simulink model "Grading_SL_Topic2"  (R2019a)
settings: Solver=FixedStepDiscrete  StartTime=0.0  StopTime=10.0  RelTol=1e-3
settings Model: Creator=Raouf  LastModifiedBy=Raouf
settings OptimizationCC: DefaultParameterBehavior=Inlined  EnhancedBackFolding=on  PassReuseOutputArgsAs=Individual arguments  OptimizeBlockOrder=speed  DifferentSizesBufferReuse=on  OptimizationCustomize=off
settings DebuggingCC: ParameterTunabilityLossMsg=error
settings SFSimCC: MATLABDynamicMemAlloc=off
settings RTWCC: SystemTargetFile=ert.tlc  GenCodeOnly=on  TemplateMakefile=ert_default_tmf  GenerateReport=on  IncludeHyperlinkInReport=on  LaunchReport=on  GenerateTraceInfo=on  GenerateTraceReport=on  GenerateTraceReportSl=on  GenerateTraceReportSf=on  GenerateTraceReportEml=on
settings CodeAppCC: ForceParamTrailComments=on  IgnoreCustomStorageClasses=off  OperatorAnnotations=on  SimulinkDataObjDesc=on  SFDataObjDesc=on  InsertBlockDesc=on
settings ERTTargetCC: TargetLangStandard=C99 (ISO)  GenerateSampleERTMain=on  InlinedParameterPlacement=NonHierarchical  ERTCustomFileTemplate=example_file_process.tlc

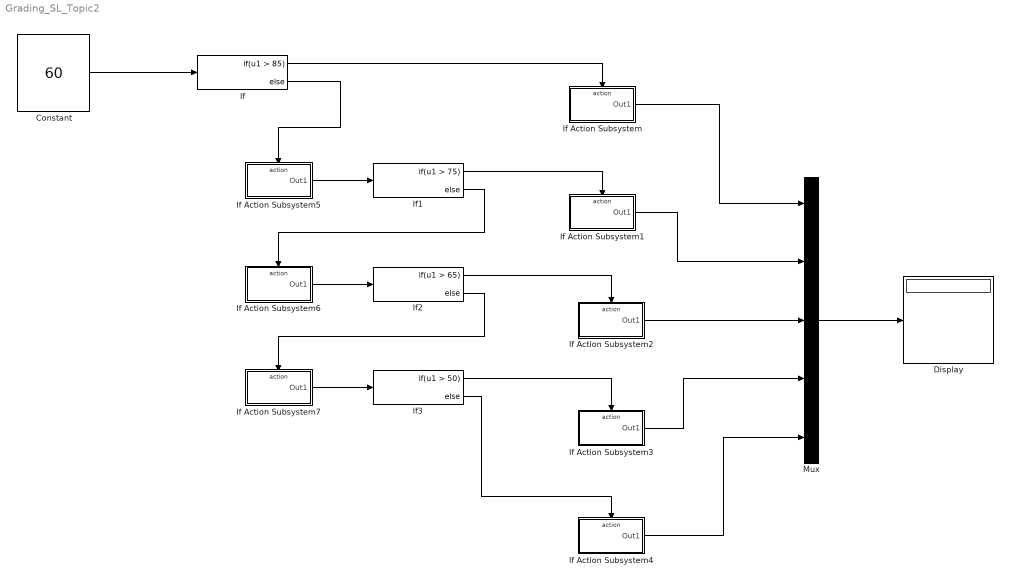
== system Grading_SL_Topic2 ==
  Constant : Constant  Value=60
  Display : Display
  If : If  IfExpression=u1 > 85
  If Action Subsystem : Subsystem  TreatAsAtomicUnit=on
  If Action Subsystem1 : Subsystem  TreatAsAtomicUnit=on
  If Action Subsystem2 : Subsystem  TreatAsAtomicUnit=on
  If Action Subsystem3 : Subsystem  TreatAsAtomicUnit=on
  If Action Subsystem4 : Subsystem  TreatAsAtomicUnit=on
  If Action Subsystem5 : Subsystem  TreatAsAtomicUnit=on
  If Action Subsystem6 : Subsystem  TreatAsAtomicUnit=on
  If Action Subsystem7 : Subsystem  TreatAsAtomicUnit=on
  If1 : If  IfExpression=u1 > 75
  If2 : If  IfExpression=u1 > 65
  If3 : If  IfExpression=u1 > 50
  Mux : Mux  Inputs=5
  wires:
  Constant/1 -> If/1
  If/1 -> If Action Subsystem/Action
  If1/1 -> If Action Subsystem1/Action
  If2/1 -> If Action Subsystem2/Action
  If3/1 -> If Action Subsystem3/Action
  If3/2 -> If Action Subsystem4/Action
  If Action Subsystem/1(Out1) -> Mux/1
  If Action Subsystem1/1(Out1) -> Mux/2
  If Action Subsystem2/1(Out1) -> Mux/3
  If Action Subsystem3/1(Out1) -> Mux/4
  If Action Subsystem4/1(Out1) -> Mux/5
  Mux/1 -> Display/1
  If/2 -> If Action Subsystem5/Action
  If Action Subsystem5/1(Out1) -> If1/1
  If1/2 -> If Action Subsystem6/Action
  If Action Subsystem6/1(Out1) -> If2/1
  If2/2 -> If Action Subsystem7/Action
  If Action Subsystem7/1(Out1) -> If3/1

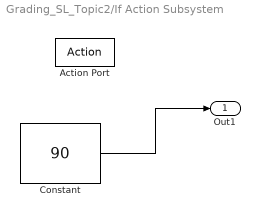
== system Grading_SL_Topic2/If Action Subsystem ==
  Action Port : ActionPort  ActionPortLabel=if(u1 > 85)
  Constant : Constant  Value=90
  Out1 : Outport
  wires:
  Constant/1 -> Out1/1

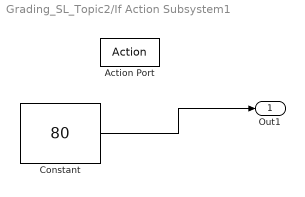
== system Grading_SL_Topic2/If Action Subsystem1 ==
  Action Port : ActionPort  ActionPortLabel=if(u1 > 75)
  Constant : Constant  Value=80
  Out1 : Outport
  wires:
  Constant/1 -> Out1/1

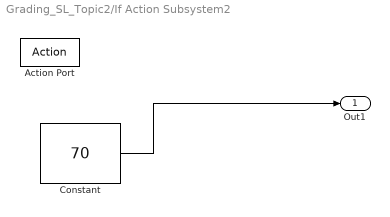
== system Grading_SL_Topic2/If Action Subsystem2 ==
  Action Port : ActionPort  ActionPortLabel=if(u1 > 65)
  Constant : Constant  Value=70
  Out1 : Outport
  wires:
  Constant/1 -> Out1/1

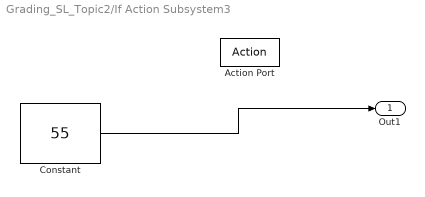
== system Grading_SL_Topic2/If Action Subsystem3 ==
  Action Port : ActionPort  ActionPortLabel=if(u1 > 50)
  Constant : Constant  Value=55
  Out1 : Outport
  wires:
  Constant/1 -> Out1/1

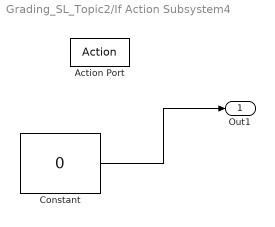
== system Grading_SL_Topic2/If Action Subsystem4 ==
  Action Port : ActionPort  ActionPortLabel=else
  Constant : Constant  Value=0
  Out1 : Outport
  wires:
  Constant/1 -> Out1/1

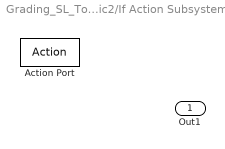
== system Grading_SL_Topic2/If Action Subsystem5 ==
  Action Port : ActionPort  ActionPortLabel=else
  Out1 : Outport

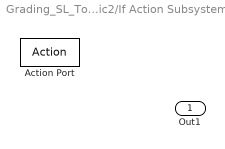
== system Grading_SL_Topic2/If Action Subsystem6 ==
  Action Port : ActionPort  ActionPortLabel=else
  Out1 : Outport

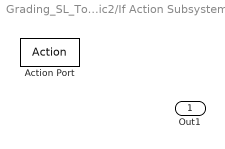
== system Grading_SL_Topic2/If Action Subsystem7 ==
  Action Port : ActionPort  ActionPortLabel=else
  Out1 : Outport
